simulink model "lab2_4_state_feed"  (R2023a)
settings: Solver=VariableStepAuto  StartTime=0.0  StopTime=2  RelTol=1e-3
values from neighbouring files (symbols this model uses):
  A = eye(3) + Ts * A    [part_deriv.m]
undefined symbols (not defined in the file or in its folder): B, K, u0, x10, x20, x30
settings Model: Creator=bz  LastModifiedBy=bz

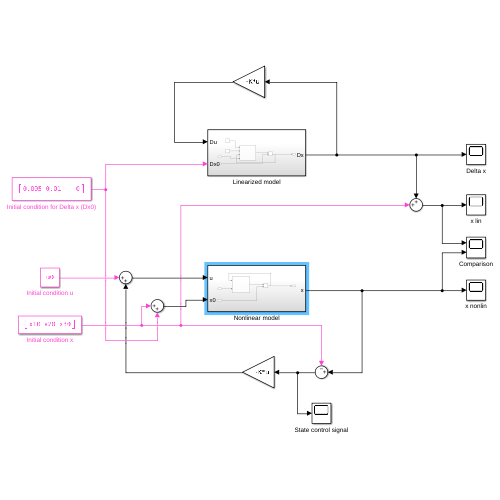
[thumbnail: Simulink's stored preview of the top-level diagram]
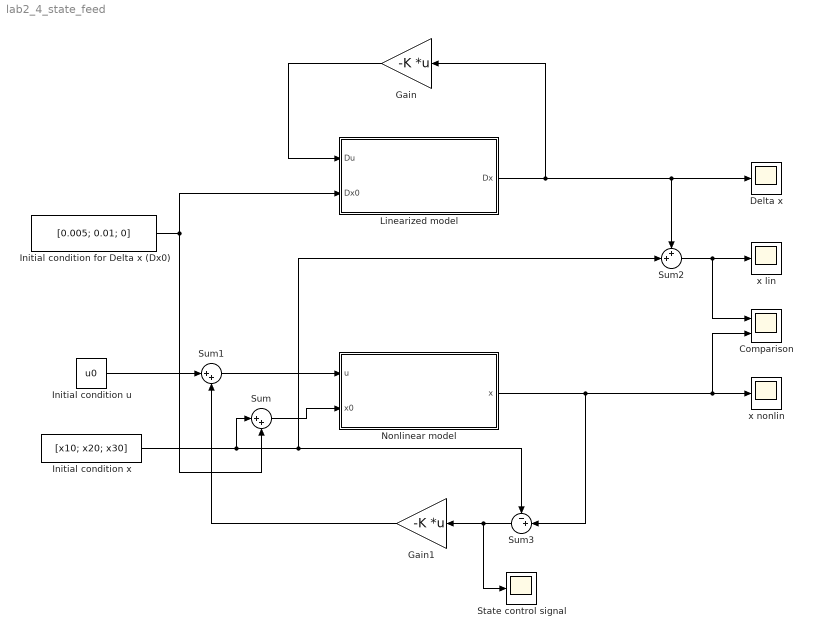
== system lab2_4_state_feed ==
  Comparison : Scope  NumInputPorts=2
  Delta x : Scope
  Gain : Gain  Gain=-K  Multiplication=Matrix(K*u)
  Gain1 : Gain  Gain=-K  Multiplication=Matrix(K*u)
  Initial condition for Delta x (Dx0) : Constant  Value=[0.005; 0.01; 0]
  Initial condition u : Constant  Value=u0
  Initial condition x : Constant  Value=[x10; x20; x30]
  Linearized model : Subsystem
  Nonlinear model : Subsystem
  State control signal : Scope
  Sum : Sum  Inputs=|++
  Sum1 : Sum  Inputs=|++
  Sum2 : Sum  Inputs=++|
  Sum3 : Sum  Inputs=-+|
  x lin : Scope
  x nonlin : Scope
  wires:
  Initial condition for Delta x (Dx0)/1 -> Sum/2, Linearized model/2(Dx0)
  Initial condition x/1 -> Sum3/1, Sum2/2, Sum/1
  Sum2/1 -> Comparison/1, x lin/1
  Linearized model/1(Dx) -> Gain/1, Delta x/1, Sum2/1
  Sum1/1 -> Nonlinear model/1(u)
  Sum/1 -> Nonlinear model/2(x0)
  Nonlinear model/1(x) -> Sum3/2, Comparison/2, x nonlin/1
  Gain/1 -> Linearized model/1(Du)
  Initial condition u/1 -> Sum1/1
  Sum3/1 -> State control signal/1, Gain1/1
  Gain1/1 -> Sum1/2

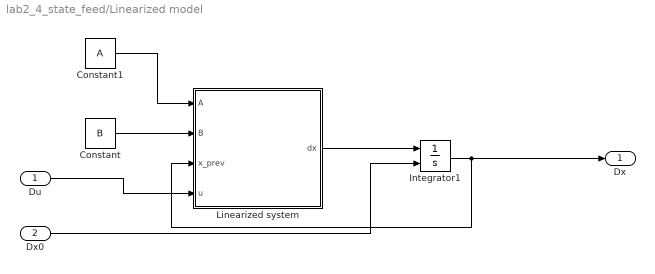
== system lab2_4_state_feed/Linearized model ==
  Du : Inport
  Dx0 : Inport  Port=2
  Constant : Constant  Value=B
  Constant1 : Constant  Value=A
  Integrator1 : Integrator  InitialConditionSource=external
  Linearized system : MATLAB Function  TreatAsAtomicUnit=on
  Dx : Outport
  wires:
  Linearized system/1(dx) -> Integrator1/1
  Integrator1/1 -> Dx/1, Linearized system/3(x_prev)
  Dx0/1 -> Integrator1/2
  Du/1 -> Linearized system/4(u)
  Constant1/1 -> Linearized system/1(A)
  Constant/1 -> Linearized system/2(B)

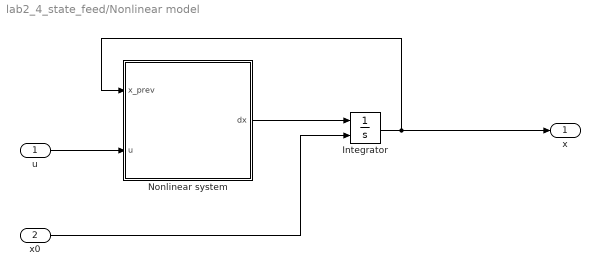
== system lab2_4_state_feed/Nonlinear model ==
  u : Inport
  x0 : Inport  Port=2
  Integrator : Integrator  InitialConditionSource=external
  Nonlinear system : MATLAB Function  TreatAsAtomicUnit=on
  x : Outport
  wires:
  Integrator/1 -> x/1, Nonlinear system/1(x_prev)
  Nonlinear system/1(dx) -> Integrator/1
  x0/1 -> Integrator/2
  u/1 -> Nonlinear system/2(u)

== matlab function lab2_4_state_feed/Linearized model/Linearized system ==
  data: A input; B input; x_prev input; u input; dx output size=[3,1]
function dx  = fcn(A, B, x_prev, u)


dx = A * x_prev + B * u;

end

== matlab function lab2_4_state_feed/Nonlinear model/Nonlinear system ==
  data: x_prev input; u input; dx output size=[3,1]
function dx  = fcn(x_prev, u)

x1 = x_prev(1);
x2 = x_prev(2);
x3 = x_prev(3);

FemP1 = 0.017521;
FemP2 = 0.0058231;

ci = -0.4;
ki = 4.4;
m = 0.016;
g = 9.81;

fiP1 = 1.4142e-4;
fiP2 = 4.5626e-3;

x1_dot = x2;
x2_dot = -(x3^2)*(FemP1/(FemP2*2*m))*exp(-x1/FemP2)+g;
x3_dot = 1/((fiP1/fiP2)*exp(-x1/fiP2))*(ki*u+ci-x3);


dx = [x1_dot; x2_dot; x3_dot];

end
